simulink model "sampleModel108"  (R2021b)
settings: Solver=VariableStepAuto  StartTime=0.0  StopTime=10.0  RelTol=1e-3
undefined symbols (not defined in the file or in its folder): DiscIntNeverNeededParam, Newton, Raphson
libraries: simulink x9, slpidlib x1
settings Model: Creator=user  LastModifiedBy=user

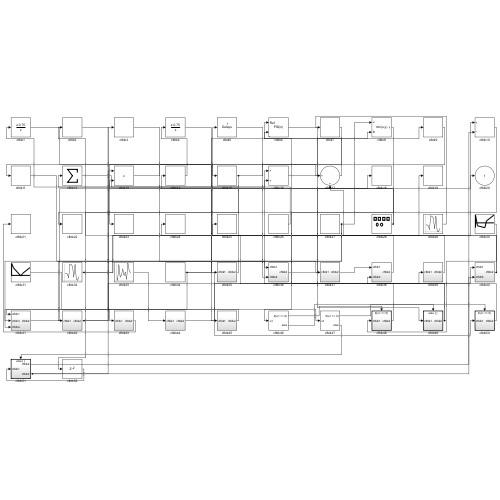
[thumbnail: Simulink's stored preview of the top-level diagram]
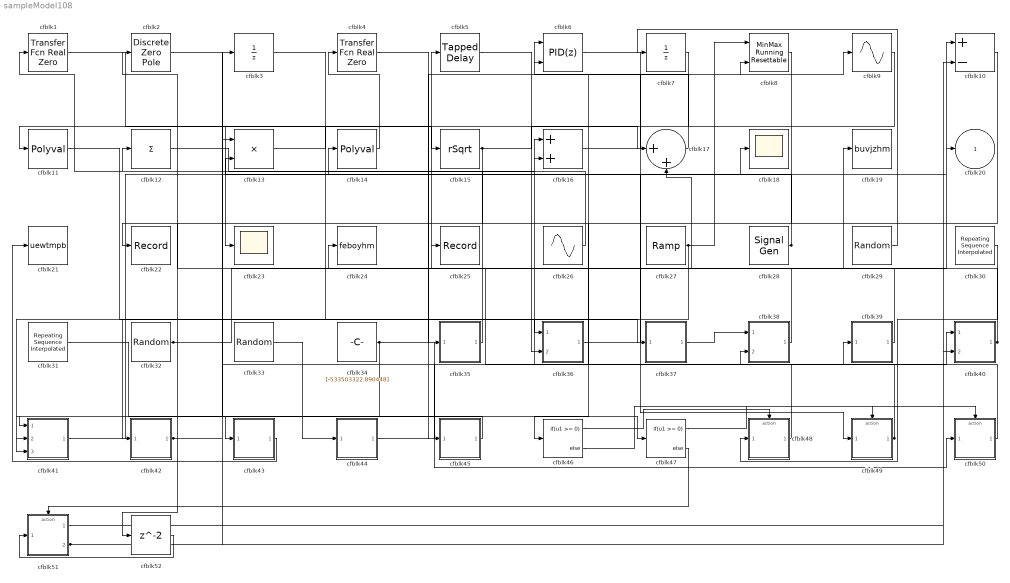
== system sampleModel108 ==
  cfblk1 : simulink/Discrete/Transfer Fcn Real Zero  ZeroZ=0.75  ICPrevInput=0.0  DoSatur=off
      settings: SourceProductBaseCode=SL
  cfblk10 : Sum  Inputs=+-
  cfblk11 : Polyval  Coefs=[ +2.081618890e-019, -1.441693666e-014, +4.719686976e-010, -8.536869453e-006, +1.621573104e-001, -8.087801117e+001 ]
  cfblk12 : Sum  Inputs=+
  cfblk13 : Product  Inputs=**
  cfblk14 : Polyval  Coefs=[ +2.081618890e-019, -1.441693666e-014, +4.719686976e-010, -8.536869453e-006, +1.621573104e-001, -8.087801117e+001 ]
  cfblk15 : Sqrt  Operator=rSqrt  AlgorithmType=Newton-Raphson  SaturateOnIntegerOverflow=on
  cfblk16 : Sum
  cfblk17 : Sum  Inputs=|++
  cfblk18 : Scope
  cfblk19 : ToWorkspace  VariableName=buvjzhm  SaveFormat=Timeseries  SampleTime=-1
  cfblk2 : DiscreteZeroPole  Poles=[0 0.5]  Gain=1
  cfblk21 : ToWorkspace  VariableName=uewtmpb  SaveFormat=Timeseries  SampleTime=-1
  cfblk22 : Record  FileSettingsInternal="{\"entries\":[{\"content\":{\"excelSettings\":{\"content\":{},\"type\":\"Streamout.ExcelSettings\"}},\"type\":\"Streamout.FileSettingStorage\",\"uuid\":\"001b1c03-1b9a-4206-ba14-e1a65e2b6dee\"}],\"packageUris\":[\"http://schema.mathworks.com/mf0/streamout_blocks/R2020a\"],\"version\":\"1.0\"}"  SignalsInternal="{\"entries\":[{\"content\":{\"signals\":[{\"content\":{\"blockPath\":[\"sampleModel108/cfblk22\"],\"channel\":[],\"dimensions\":[1],\"domain\":\"sampleModel108/cfblk22\",\"lineColor\":\"#edb120\",\"plots\":[1],\"port\":1,\"sid\":[\"\"],\"signalID\":3819,\"signalName\":\"cfblk15\"},\"type\":\"RecordBlkView.Signal\",\"uuid\":\"c14f24dc-517d-4b14-9c6c-5f234a6a3d35\"}]},\"type\":\"RecordBlkView.InputSignals\",\"uuid\":\"03286de0-e967-40d7-b892-a908d484ed90\"}],\"packageUris\":[\"http://schema.mathworks.com/mf0/streamout_blocks/R2020a\"],\"version\":\"1.0\"}"  VisualizationBindings="{\"sparklinesplugin\":{\"info\":[{\"bindingParametersList\":[],\"subplotID\":1}]}}"
  cfblk23 : Scope
  cfblk24 : ToWorkspace  VariableName=feboyhm  SaveFormat=Timeseries  SampleTime=-1
  cfblk25 : Record  FileSettingsInternal="{\"entries\":[{\"content\":{\"excelSettings\":{\"content\":{},\"type\":\"Streamout.ExcelSettings\"}},\"type\":\"Streamout.FileSettingStorage\",\"uuid\":\"abbdaaeb-bfa7-4130-ae6d-2dc964ecb0b2\"}],\"packageUris\":[\"http://schema.mathworks.com/mf0/streamout_blocks/R2020a\"],\"version\":\"1.0\"}"  SignalsInternal="{\"entries\":[{\"content\":{\"signals\":[{\"content\":{\"blockPath\":[\"sampleModel108/cfblk25\"],\"channel\":[],\"dimensions\":[1],\"domain\":\"sampleModel108/cfblk25\",\"lineColor\":\"#7e2f8e\",\"plots\":[1],\"port\":1,\"sid\":[\"\"],\"signalID\":3823,\"signalName\":\"cfblk50\"},\"type\":\"RecordBlkView.Signal\",\"uuid\":\"64a622d0-8ad5-4104-894f-c9aafd74877a\"}]},\"type\":\"RecordBlkView.InputSignals\",\"uuid\":\"17d718b0-2577-4f4e-ad25-bdc57ca26761\"}],\"packageUris\":[\"http://schema.mathworks.com/mf0/streamout_blocks/R2020a\"],\"version\":\"1.0\"}"  VisualizationBindings="{\"sparklinesplugin\":{\"info\":[{\"bindingParametersList\":[],\"subplotID\":1}]}}"
  cfblk26 : Sin  Amplitude=[-496472036.710495]  Bias=[-359639312.603698]  SampleTime=0
  cfblk27 : simulink/Sources/Ramp  slope=[2265.952961]  start=[37.084199]  InitialOutput=[982752.553315]
  cfblk28 : SignalGenerator  WaveForm=sawtooth  Amplitude=[-960338777.696214]
  cfblk29 : RandomNumber  Mean=[-66230.144972]  Variance=[94247.145385]  Seed=[238155845.000000]  SampleTime=0.1
  cfblk3 : UnitDelay  HasFrameUpgradeWarning=on
  cfblk30 : simulink/Sources/Repeating Sequence Interpolated  OutValues=[871981444.876662, -319162565.924685, -506350222.551510, 237134094.361118, 849934068.477172]  TimeValues=[0 0.1 0.5 0.6 1].'  LookUpMeth=Use Input Below  tsamp=0.01  OutMin=[]  OutMax=[]  OutDataTypeStr=double  OutputDataTypeScalingMode=double  OutDataType=fixdt(0,8)  OutScaling=2^-10
  cfblk31 : simulink/Sources/Repeating Sequence Interpolated  OutValues=[958364184.959801, 604286849.411846, -34917419.882751, 173210394.411302, 619436100.017050]  TimeValues=[0 0.1 0.5 0.6 1].'  LookUpMeth=Use Input Nearest  tsamp=0.01  OutMin=[]  OutMax=[]  OutDataTypeStr=double  OutputDataTypeScalingMode=double  OutDataType=fixdt(0,8)  OutScaling=2^-10
  cfblk32 : RandomNumber  Mean=[31789.555588]  Variance=[61002.776115]  Seed=[547000665.000000]  SampleTime=0.1
  cfblk33 : UniformRandomNumber  Minimum=[-7974569136.520132]  Maximum=[5305807397.560600]  Seed=[57992090.000000]  SampleTime=0.1
  cfblk34 : Constant  Value=[-533503322.890448]  SampleTime=1
  cfblk35 : Subsystem
  cfblk36 : Subsystem
  cfblk37 : Subsystem
  cfblk38 : Subsystem
  cfblk39 : Subsystem
  cfblk4 : simulink/Discrete/Transfer Fcn Real Zero  ZeroZ=0.75  ICPrevInput=0.0  DoSatur=off
      settings: SourceProductBaseCode=SL
  cfblk40 : Subsystem
  cfblk41 : Subsystem
  cfblk42 : Subsystem
  cfblk43 : Subsystem
  cfblk44 : Subsystem
  cfblk45 : Subsystem
  cfblk46 : If  IfExpression=u1 >= 0  SampleTime=1
  cfblk47 : If  IfExpression=u1 >= 0  SampleTime=1
  cfblk48 : Subsystem  TreatAsAtomicUnit=on
  cfblk49 : Subsystem  TreatAsAtomicUnit=on
  cfblk5 : simulink/Discrete/Tapped Delay  vinit=0.0  samptime=-1  NumDelays=1  DelayOrder=Oldest  includeCurrent=off
  cfblk50 : Subsystem  TreatAsAtomicUnit=on
  cfblk51 : Subsystem  TreatAsAtomicUnit=on
  cfblk52 : Delay  SampleTime=1
  cfblk6 : slpidlib/PID Controller (2DOF)  Controller=PID  Form=Parallel  TimeDomain=Discrete-time  UseExternalTs=off  SampleTime=1  IntegratorMethod=Forward Euler  FilterMethod=Forward Euler  ControllerParametersSource=internal  P=1  I=1  D=0  UseFilter=on  N=100  b=1  c=1  TunerSelectOption=Transfer Function Based (PID Tuner App)  InitialConditionSource=internal  InitialConditionForIntegrator=0  InitialConditionForFilter=0  DifferentiatorICPrevScaledInput=0  ExternalReset=none  TrackingMode=off  Kt=1  LimitOutput=off  SatLimitsSource=internal  UpperSaturationLimit=inf  LowerSaturationLimit=-inf  LinearizeAsGain=off  AntiWindupMode=none  Kb=1  POutMin=[]  POutMax=[]  IOutMin=[]  IOutMax=[]  DOutMin=[]  DOutMax=[]  NOutMin=[]  NOutMax=[]  bOutMin=[]  bOutMax=[]  cOutMin=[]  cOutMax=[]  SumOutMin=[]  SumOutMax=[]  SaturationOutMin=[]  SaturationOutMax=[]  PParamMin=[]  PParamMax=[]  IParamMin=[]  IParamMax=[]  DParamMin=[]  DParamMax=[]  NParamMin=[]  NParamMax=[]  bParamMin=[]  bParamMax=[]  cParamMin=[]  cParamMax=[]  KbParamMin=[]  KbParamMax=[]  KtParamMin=[]  KtParamMax=[]  KbOutMin=[]  KbOutMax=[]  KtOutMin=[]  KtOutMax=[]  IntegratorOutMin=[]  IntegratorOutMax=[]  FilterOutMin=[]  FilterOutMax=[]  SumI1OutMin=[]  SumI1OutMax=[]  SumI2OutMin=[]  SumI2OutMax=[]  SumI3OutMin=[]  SumI3OutMax=[]  SumI4OutMin=[]  SumI4OutMax=[]  SumDOutMin=[]  SumDOutMax=[]  Sum1OutMin=[]  Sum1OutMax=[]  Sum2OutMin=[]  Sum2OutMax=[]  Sum3OutMin=[]  Sum3OutMax=[]  DifferentiatorOutMin=[]  DifferentiatorOutMax=[]  FilterDiffOutCoefMin=[]  FilterDiffOutCoefMax=[]  ReciprocalOutMin=[]  ReciprocalOutMax=[]  SumDenOutMin=[]  SumDenOutMax=[]  SumNumOutMin=[]  SumNumOutMax=[]  DivideOutMin=[]  DivideOutMax=[]  UdiffTsProdOutMin=[]  UdiffTsProdOutMax=[]  NTsProdOutMin=[]  NTsProdOutMax=[]  UintegralTsProdOutMin=[]  UintegralTsProdOutMax=[]  UngainTsProdOutMin=[]  UngainTsProdOutMax=[]  IntegratorContinuousStateAttributes=''  IntegratorStateMustResolveToSignalObject=off  IntegratorRTWStateStorageClass=Auto  FilterContinuousStateAttributes=''  FilterStateMustResolveToSignalObject=off  FilterRTWStateStorageClass=Auto  ParallelPVariant=InternalParameters  IdealPVariant=Disabled  IVariant=InternalParameters  DVariant=InternalParameters  bVariant=InternalParameters  cVariant=InternalParameters  IntegratorVariant=Discrete  SatVariant=Disabled  AWVariant=Passthrough  PCopyVariant=Disabled  TRVariant=Disabled  FdbkBlocksVariant=Forward  IdealPFdbkVariant=Disabled  SatFdbkVariant=Disabled  DerivativeFilterVariant=ForwardEulerFilter  NVariant=InternalParameters  NCopyVariant=Disabled  FilterICVariant=InternalICsFilter  IntegratorICVariant=InternalICs  ExternalResetVariant=Disabled  TRSumVariant=Passthrough  SumFdbkVariant=Disabled  SumVariant=Sum_PID  TsampFilterVariant=InternalTs  TsampNgainVariant=Passthrough  TsampIntegralVariant=Passthrough  ExternalSaturationOutDataTypeStr=Inherit: Same as second input
      settings: SourceProductBaseCode=SL
  cfblk7 : UnitDelay  HasFrameUpgradeWarning=on
  cfblk8 : simulink/Math Operations/MinMax Running Resettable  Function=min  vinit=0.0
  cfblk9 : Sin  TimeSource=Use external signal  SampleTime=0
  cfblk20 : Outport
  wires:
  cfblk31/1 -> cfblk43/1(cfblk1)
  cfblk9/1 -> cfblk11/1
  cfblk35/1(cfblk2) -> cfblk12/1
  cfblk14/1 -> cfblk4/1
  cfblk28/1 -> cfblk14/1, cfblk13/2
  cfblk42/1(cfblk2) -> cfblk3/1, cfblk40/1(cfblk1)
  cfblk49/1(cfblk2) -> cfblk16/1, cfblk38/2(cfblk3)
  cfblk30/1 -> cfblk48/1(cfblk1)
  cfblk41/1(cfblk2) -> cfblk18/1
  cfblk34/1 -> cfblk50/1(cfblk1), cfblk8/2, cfblk41/3(cfblk4)
  cfblk40/1(cfblk2) -> cfblk5/1, cfblk17/2
  cfblk38/1(cfblk2) -> cfblk24/1
  cfblk6/1 -> cfblk49/1(cfblk1)
  cfblk29/1 -> cfblk7/1
  cfblk32/1 -> cfblk10/1, cfblk19/1
  cfblk33/1 -> cfblk44/1(cfblk1)
  cfblk7/1 -> cfblk23/1
  cfblk13/1 -> cfblk15/1
  cfblk45/1(cfblk2) -> cfblk41/1(cfblk1)
  cfblk1/1 -> cfblk35/1(cfblk1)
  cfblk36/1(cfblk2) -> cfblk20/1
  cfblk39/1(cfblk2) -> cfblk2/1
  cfblk3/1 -> cfblk36/1(cfblk1)
  cfblk5/1 -> cfblk36/2(cfblk4)
  cfblk43/1(cfblk2) -> cfblk21/1
  cfblk12/1 -> cfblk16/2
  cfblk26/1 -> cfblk1/1
  cfblk51/1(cfblk2) -> cfblk10/2
  cfblk17/1 -> cfblk6/1
  cfblk48/1(cfblk2) -> cfblk6/2
  cfblk51/2(cfblk3) -> cfblk13/1, cfblk40/2(cfblk5)
  cfblk15/1 -> cfblk22/1, cfblk17/1
  cfblk8/1 -> cfblk46/1
  cfblk44/1(cfblk2) -> cfblk39/1(cfblk1)
  cfblk16/1 -> cfblk9/1
  cfblk27/1 -> cfblk42/1(cfblk1), cfblk8/1, cfblk41/2(cfblk3)
  cfblk37/1(cfblk2) -> cfblk38/1(cfblk1)
  cfblk2/1 -> cfblk47/1
  cfblk4/1 -> cfblk45/1(cfblk1)
  cfblk11/1 -> cfblk37/1(cfblk1)
  cfblk50/1(cfblk2) -> cfblk25/1
  cfblk46/1 -> cfblk48/Action
  cfblk46/2 -> cfblk49/Action
  cfblk47/1 -> cfblk50/Action
  cfblk47/2 -> cfblk51/Action
  cfblk10/1 -> cfblk52/1
  cfblk52/1 -> cfblk51/1(cfblk1)

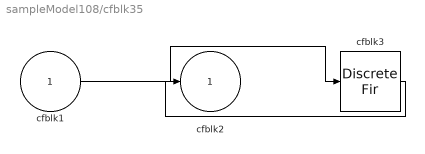
== system sampleModel108/cfblk35 ==
  cfblk1 : Inport
  cfblk3 : DiscreteFir  SampleTime=1
  cfblk2 : Outport
  wires:
  cfblk1/1 -> cfblk3/1
  cfblk3/1 -> cfblk2/1

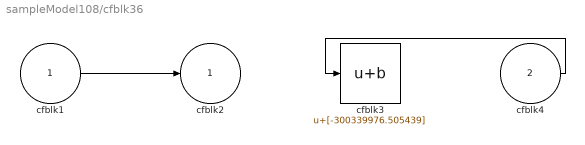
== system sampleModel108/cfblk36 ==
  cfblk1 : Inport
  cfblk4 : Inport  Port=2
  cfblk3 : Bias  Bias=[-300339976.505439]
  cfblk2 : Outport
  wires:
  cfblk1/1 -> cfblk2/1
  cfblk4/1 -> cfblk3/1

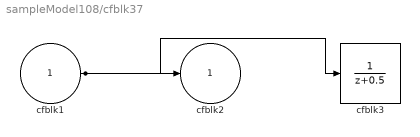
== system sampleModel108/cfblk37 ==
  cfblk1 : Inport
  cfblk3 : DiscreteTransferFcn  SampleTime=1
  cfblk2 : Outport
  wires:
  cfblk1/1 -> cfblk2/1, cfblk3/1

== system sampleModel108/cfblk38 ==
  cfblk1 : Inport
  cfblk3 : Inport  Port=2
  cfblk2 : Outport
  wires:
  cfblk3/1 -> cfblk2/1

== system sampleModel108/cfblk39 ==
  cfblk1 : Inport
  cfblk3 : DiscreteIntegrator  ICPrevOutput=DiscIntNeverNeededParam  ICPrevScaledInput=DiscIntNeverNeededParam
  cfblk2 : Outport
  wires:
  cfblk3/1 -> cfblk2/1
  cfblk1/1 -> cfblk3/1

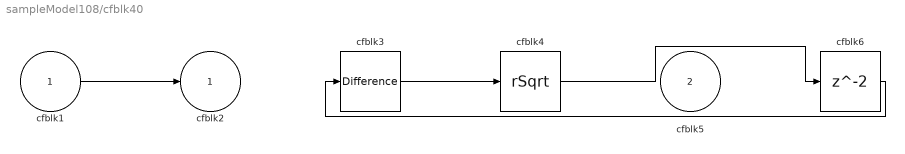
== system sampleModel108/cfblk40 ==
  cfblk1 : Inport
  cfblk5 : Inport  Port=2
  cfblk3 : simulink/Discrete/Difference  ICPrevInput=0.0  OutMin=[]  OutMax=[]  OutDataTypeStr=Inherit: Inherit via back propagation  OutDataType=fixdt(1, 16)  OutScaling=2^-10  DoSatur=off
  cfblk4 : Sqrt  Operator=rSqrt  AlgorithmType=Newton-Raphson  SaturateOnIntegerOverflow=on
  cfblk6 : Delay  SampleTime=1
  cfblk2 : Outport
  wires:
  cfblk3/1 -> cfblk4/1
  cfblk1/1 -> cfblk2/1
  cfblk4/1 -> cfblk6/1
  cfblk6/1 -> cfblk3/1

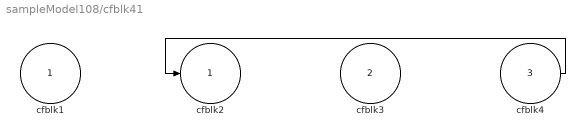
== system sampleModel108/cfblk41 ==
  cfblk1 : Inport
  cfblk3 : Inport  Port=2
  cfblk4 : Inport  Port=3
  cfblk2 : Outport
  wires:
  cfblk4/1 -> cfblk2/1

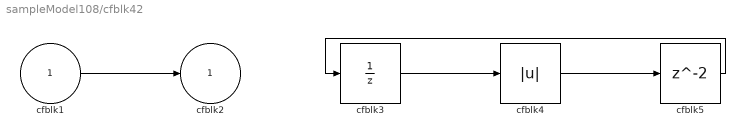
== system sampleModel108/cfblk42 ==
  cfblk1 : Inport
  cfblk3 : UnitDelay  HasFrameUpgradeWarning=on
  cfblk4 : Abs
  cfblk5 : Delay  SampleTime=1
  cfblk2 : Outport
  wires:
  cfblk1/1 -> cfblk2/1
  cfblk3/1 -> cfblk4/1
  cfblk4/1 -> cfblk5/1
  cfblk5/1 -> cfblk3/1

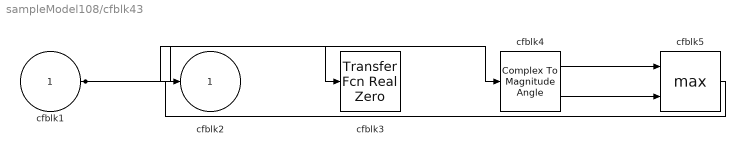
== system sampleModel108/cfblk43 ==
  cfblk1 : Inport
  cfblk3 : simulink/Discrete/Transfer Fcn Real Zero  ZeroZ=0.75  ICPrevInput=0.0  DoSatur=off
      settings: SourceProductBaseCode=SL
  cfblk4 : ComplexToMagnitudeAngle
  cfblk5 : MinMax  Function=max  Inputs=2
  cfblk2 : Outport
  wires:
  cfblk4/1 -> cfblk5/1
  cfblk1/1 -> cfblk4/1, cfblk3/1
  cfblk4/2 -> cfblk5/2
  cfblk5/1 -> cfblk2/1

== system sampleModel108/cfblk44 ==
  cfblk1 : Inport
  cfblk3 : DiscreteIntegrator  ICPrevOutput=DiscIntNeverNeededParam  ICPrevScaledInput=DiscIntNeverNeededParam
  cfblk2 : Outport
  wires:
  cfblk1/1 -> cfblk3/1
  cfblk3/1 -> cfblk2/1

== system sampleModel108/cfblk45 ==
  cfblk1 : Inport
  cfblk3 : Constant  Value=[765944321.386147]  SampleTime=1
  cfblk2 : Outport
  wires:
  cfblk3/1 -> cfblk2/1

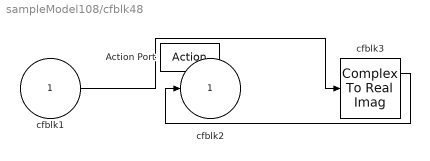
== system sampleModel108/cfblk48 ==
  cfblk1 : Inport
  Action Port : ActionPort  ActionPortLabel=if(u1 >= 0)
  cfblk3 : ComplexToRealImag
  cfblk2 : Outport
  wires:
  cfblk3/1 -> cfblk2/1
  cfblk1/1 -> cfblk3/1

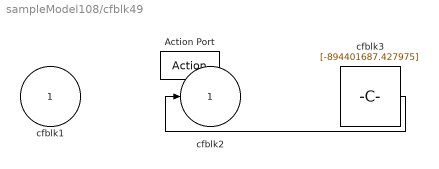
== system sampleModel108/cfblk49 ==
  cfblk1 : Inport
  Action Port : ActionPort  ActionPortLabel=else
  cfblk3 : Constant  Value=[-894401687.427975]  SampleTime=1
  cfblk2 : Outport
  wires:
  cfblk3/1 -> cfblk2/1

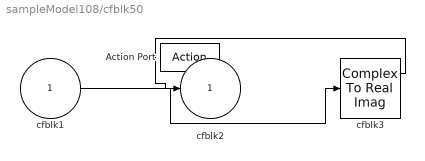
== system sampleModel108/cfblk50 ==
  cfblk1 : Inport
  Action Port : ActionPort  ActionPortLabel=if(u1 >= 0)
  cfblk3 : ComplexToRealImag
  cfblk2 : Outport
  wires:
  cfblk1/1 -> cfblk3/1
  cfblk3/1 -> cfblk2/1

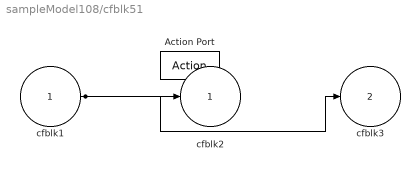
== system sampleModel108/cfblk51 ==
  cfblk1 : Inport
  Action Port : ActionPort  ActionPortLabel=else
  cfblk2 : Outport
  cfblk3 : Outport  Port=2
  wires:
  cfblk1/1 -> cfblk2/1, cfblk3/1
